simulink model "sub_system"  (R2020a)
settings: Solver=VariableStepAuto  StartTime=0.0  StopTime=10.0  RelTol=1e-3
settings Model: Creator=Administrator  LastModifiedBy=Administrator

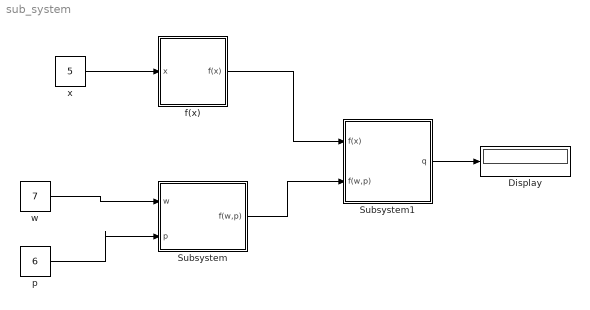
== system sub_system ==
  Display : Display
  Subsystem : Subsystem
  Subsystem1 : Subsystem
  f(x) : Subsystem
  p : Constant  Value=6
  w : Constant  Value=7
  x : Constant  Value=5
  wires:
  x/1 -> f(x)/1(x)
  w/1 -> Subsystem/1(w)
  p/1 -> Subsystem/2(p)
  Subsystem/1(f(w,p)) -> Subsystem1/2(f(w,p))
  f(x)/1(f(x)) -> Subsystem1/1(f(x))
  Subsystem1/1(q) -> Display/1

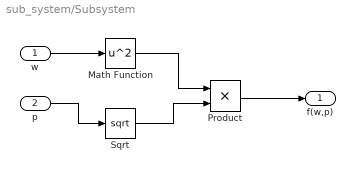
== system sub_system/Subsystem ==
  w : Inport
  p : Inport  Port=2
  Math Function : Math  Operator=square  SaturateOnIntegerOverflow=on
  Product : Product
  Sqrt : Sqrt  SaturateOnIntegerOverflow=on
  f(w,p) : Outport
  wires:
  w/1 -> Math Function/1
  Product/1 -> f(w,p)/1
  Sqrt/1 -> Product/2
  Math Function/1 -> Product/1
  p/1 -> Sqrt/1

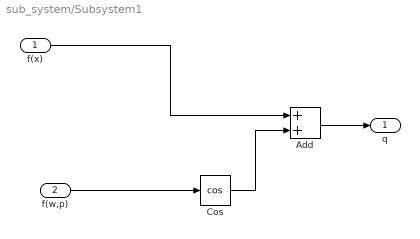
== system sub_system/Subsystem1 ==
  f(x) : Inport
  f(w,p) : Inport  Port=2
  Add : Sum
  Cos : Trigonometry  Operator=cos
  q : Outport
  wires:
  Add/1 -> q/1
  Cos/1 -> Add/2
  f(x)/1 -> Add/1
  f(w,p)/1 -> Cos/1

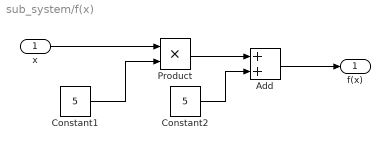
== system sub_system/f(x) ==
  x : Inport
  Add : Sum
  Constant1 : Constant  Value=5
  Constant2 : Constant  Value=5
  Product : Product
  f(x) : Outport
  wires:
  Product/1 -> Add/1
  x/1 -> Product/1
  Constant1/1 -> Product/2
  Add/1 -> f(x)/1
  Constant2/1 -> Add/2
